simulink model "output"  (R2016b)
settings: Solver=VariableStepAuto  StartTime=0.0  StopTime=10.0  RelTol=1e-3
libraries: commutil2 x1
settings Model: Creator=张尧  LastModifiedBy=张尧

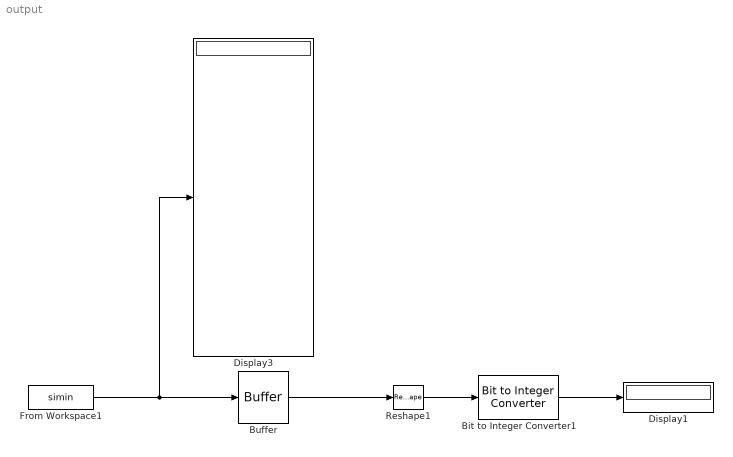
== system output ==
  Bit to Integer Converter1 : commutil2/Bit to Integer Converter  nbits=16  bitOrder=MSB first  signedOutputValues=Unsigned  outDtype=Inherit via internal rule  outDtypeSigned=Inherit via internal rule
  Buffer : Buffer  N=16  TreatMby1Signals=One channel  OutputFrames=off
  Display1 : Display
  Display3 : Display
  From Workspace1 : FromWorkspace  VariableName=simin  OutDataTypeStr=double  SampleTime=1
  Reshape1 : Reshape
  wires:
  From Workspace1/1 -> Display3/1, Buffer/1
  Buffer/1 -> Reshape1/1
  Reshape1/1 -> Bit to Integer Converter1/1
  Bit to Integer Converter1/1 -> Display1/1
